simulink model "Karplus_Strong"  (R2023b)
settings: Solver=FixedStepAuto  StartTime=0.0  StopTime=2.6  RelTol=1e-3
values from neighbouring files (symbols this model uses):
  period_sequence = normalised_period(f_s,zelda)    [main.m]
  T_s = 1/f_s    (= 6.25e-05)    [main.m]
undefined symbols (not defined in the file or in its folder): gaussian
libraries: simulink x3, dspvision x1
settings Model: CodeVerificationMode=processor-in-the-loop (pil)  Creator=andre  LastModifiedBy=andre
settings OptimizationCC: DefaultParameterBehavior=Inlined  EnhancedBackFolding=on  PassReuseOutputArgsAs=Individual arguments  ZeroExternalMemoryAtStartup=off  ZeroInternalMemoryAtStartup=off  OptimizeBlockOrder=speed  DifferentSizesBufferReuse=on  OptimizationCustomize=off  EfficientTunableParamExpr=on
settings DebuggingCC: ParameterTunabilityLossMsg=error
settings SFSimCC: MATLABDynamicMemAlloc=off
settings RTWCC: Description=Embedded Coder  SystemTargetFile=ert.tlc  TemplateMakefile=ert_default_tmf  GenerateReport=on  LaunchReport=on  CodeExecutionProfiling=on  CodeProfilingSaveOptions=AllData  CodeProfilingInstrumentation=detailed  GenerateWebview=on  GenerateCodeMetricsReport=on
settings CodeAppCC: ForceParamTrailComments=on  IgnoreCustomStorageClasses=off  OperatorAnnotations=on  SimulinkDataObjDesc=on  SFDataObjDesc=on  InsertBlockDesc=on
settings ERTTargetCC: TargetLangStandard=C99 (ISO)  GenerateSampleERTMain=on  InlinedParameterPlacement=NonHierarchical  ERTCustomFileTemplate=example_file_process.tlc

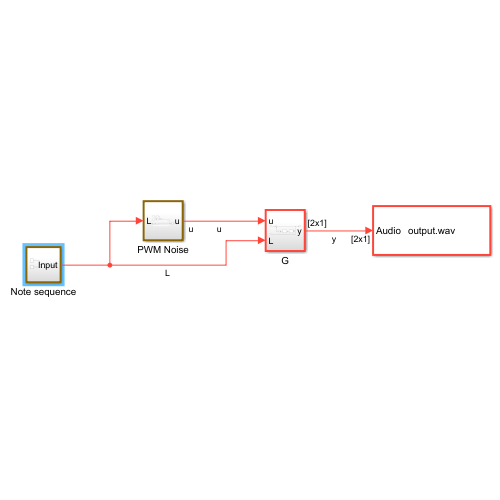
[thumbnail: Simulink's stored preview of the top-level diagram]
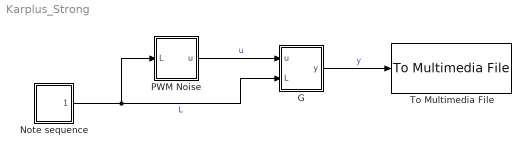
== system Karplus_Strong ==
  G : Subsystem
  Note sequence : Subsystem
  PWM Noise : Subsystem
  To Multimedia File : dspvision/To Multimedia File  outputFilename=output.wav  streamSelection=Audio only  videoCompressor=None (uncompressed)  audioCompressor=None (uncompressed)  imagePorts=Separate color signals  fileType=WAV  audioDatatype=16-bit integer  fourcc=RGB  videoQuality=75  mj2000CompFactor=10
      settings: LibrarySourceBlock=dspsnks4/To Multimedia File
  wires:
  PWM Noise/1(u) -> G/1(u)  "u"
  Note sequence/1(Input) -> PWM Noise/1(L), G/2(L)  "L"
  G/1(y) -> To Multimedia File/1  "y"

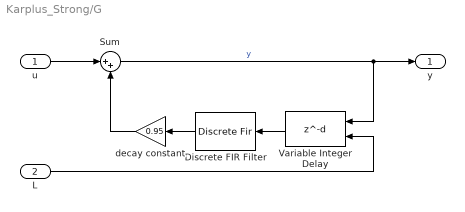
== system Karplus_Strong/G ==
  u : Inport
  L : Inport  Port=2
  Discrete FIR Filter : DiscreteFir
  Sum : Sum  Inputs=|++
  Variable Integer Delay : Delay  DelayLengthSource=Input port  DelayLengthUpperLimit=256  PreventDirectFeedthrough=on  UseCircularBuffer=on
      settings: InputPortMap=u0,p1
  decay constant : Gain  Gain=0.95
  y : Outport
  wires:
  Variable Integer Delay/1 -> Discrete FIR Filter/1
  L/1 -> Variable Integer Delay/2
  decay constant/1 -> Sum/2
  Sum/1 -> y/1, Variable Integer Delay/1  "y"
  u/1 -> Sum/1
  Discrete FIR Filter/1 -> decay constant/1

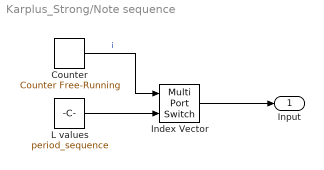
== system Karplus_Strong/Note sequence ==
  Counter : simulink/Sources/Counter Free-Running  NumBits=4  tsamp=0.2
  Index Vector : MultiPortSwitch  DataPortOrder=Zero-based contiguous  Inputs=1  zeroidx=on  SaturateOnIntegerOverflow=off  InputSameDT=off
  L values : Constant  Value=period_sequence
  Input : Outport
  wires:
  L values/1 -> Index Vector/2
  Index Vector/1 -> Input/1
  Counter/1 -> Index Vector/1  "i"

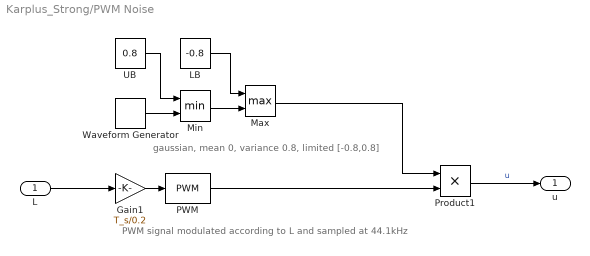
== system Karplus_Strong/PWM Noise ==
  note: PWM signal modulated according to L and sampled at 44.1kHz
  note: gaussian, mean 0, variance 0.8, limited [-0.8,0.8]
  L : Inport
  Gain1 : Gain  Gain=T_s/0.2
  LB : Constant  Value=-0.8
  Max : MinMax  Function=max  Inputs=2
  Min : MinMax  Inputs=2
  PWM : simulink/Discontinuities/PWM  DisableCoverage=on  Period=0.2  InitialDelay=0  DisallowZeroDutyCycle=off  RunAtFixedTimeIntervals=on  SampleTime=T_s
  Product1 : Product
  UB : Constant  Value=0.8
  Waveform Generator : simulink/Sources/Waveform Generator  OutMin=[]  OutMax=[]  OutDataTypeStr=double  SelectedSignal=1  Signals=gaussian('Mean',0,'Variance',0.8,'Seed',1)  BlockNames=MultiportSwitch_c96a69a61ea7450  SampleTime=T_s
  u : Outport
  wires:
  LB/1 -> Max/1
  Waveform Generator/1 -> Min/2
  UB/1 -> Min/1
  Min/1 -> Max/2
  PWM/1 -> Product1/2
  Gain1/1 -> PWM/1
  L/1 -> Gain1/1
  Product1/1 -> u/1  "u"
  Max/1 -> Product1/1
